simulink model "temp"  (R2019a)
settings: Solver=VariableStepAuto  StartTime=0.0  StopTime=10.0  RelTol=1e-3
settings Model: Creator=yahyaaba  LastModifiedBy=yahyaaba

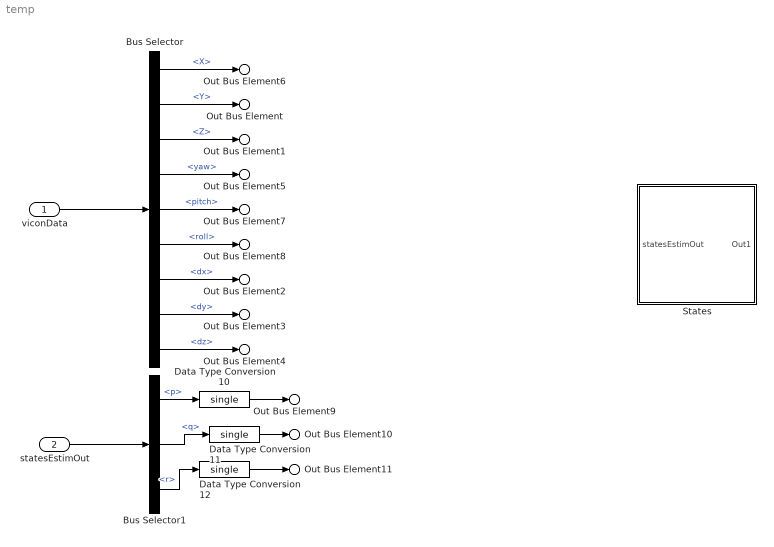
== system temp ==
  viconData : Inport  OutDataTypeStr=Bus: viconData
  statesEstimOut : Inport  Port=2
  Bus Selector : BusSelector  OutputSignals=X,Y,Z,yaw,pitch,roll,dx,dy,dz
  Bus Selector1 : BusSelector  OutputSignals=p,q,r
  Data Type Conversion10 : DataTypeConversion  OutDataTypeStr=single
  Data Type Conversion11 : DataTypeConversion  OutDataTypeStr=single
  Data Type Conversion12 : DataTypeConversion  OutDataTypeStr=single
  States : Subsystem
  Out Bus Element6 : Outport  PortName=states  Element=X
  Out Bus Element : Outport  PortName=states  Element=Y
  Out Bus Element1 : Outport  PortName=states  Element=Z
  Out Bus Element5 : Outport  PortName=states  Element=yaw
  Out Bus Element7 : Outport  PortName=states  Element=pitch
  Out Bus Element8 : Outport  PortName=states  Element=roll
  Out Bus Element2 : Outport  PortName=states  Element=dx
  Out Bus Element3 : Outport  PortName=states  Element=dy
  Out Bus Element4 : Outport  PortName=states  Element=dz
  Out Bus Element9 : Outport  PortName=states  Element=p
  Out Bus Element10 : Outport  PortName=states  Element=q
  Out Bus Element11 : Outport  PortName=states  Element=r
  wires:
  Bus Selector/4 -> Out Bus Element5/1  "<yaw>"
  Bus Selector/2 -> Out Bus Element/1  "<Y>"
  Bus Selector1/1 -> Data Type Conversion10/1  "<p>"
  Bus Selector/7 -> Out Bus Element2/1  "<dx>"
  Bus Selector/1 -> Out Bus Element6/1  "<X>"
  Bus Selector1/3 -> Data Type Conversion12/1  "<r>"
  Bus Selector/5 -> Out Bus Element7/1  "<pitch>"
  Bus Selector/6 -> Out Bus Element8/1  "<roll>"
  Bus Selector1/2 -> Data Type Conversion11/1  "<q>"
  Data Type Conversion10/1 -> Out Bus Element9/1
  Data Type Conversion12/1 -> Out Bus Element11/1
  Data Type Conversion11/1 -> Out Bus Element10/1
  statesEstimOut/1 -> Bus Selector1/1
  viconData/1 -> Bus Selector/1
  Bus Selector/8 -> Out Bus Element3/1  "<dy>"
  Bus Selector/3 -> Out Bus Element1/1  "<Z>"
  Bus Selector/9 -> Out Bus Element4/1  "<dz>"

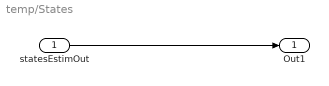
== system temp/States ==
  statesEstimOut : Inport  OutDataTypeStr=Bus: statesEstim_t
  Out1 : Outport  OutDataTypeStr=Bus: statesBB
  wires:
  statesEstimOut/1 -> Out1/1
